simulink model "time_conv_test"  (R2016b)
settings: Solver=VariableStepAuto  StartTime=0.0  StopTime=0  RelTol=1e-3
libraries: GPS_time_lib x1, YMDHMS_2_dec_year x1, time_conversion_lib x1
settings Model: Creator=Taylor  LastModifiedBy=Taylor

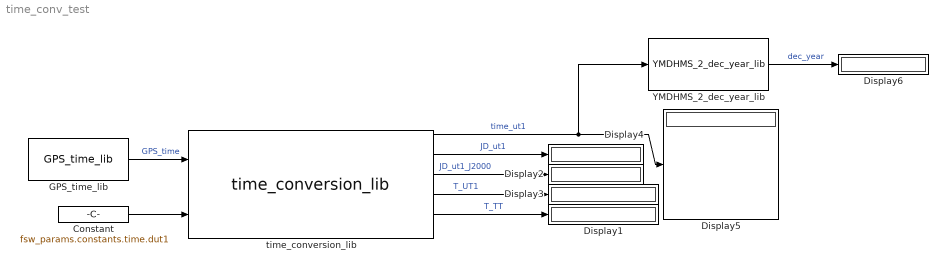
== system time_conv_test ==
  Constant : Constant  Value=fsw_params.constants.time.dut1
  Display{1..6} (6 alike) : Display
  GPS_time_lib : GPS_time_lib/GPS_time_lib
  YMDHMS_2_dec_year_lib : YMDHMS_2_dec_year/YMDHMS_2_dec_year_lib
  time_conversion_lib : time_conversion_lib/time_conversion_lib
  wires:
  GPS_time_lib/1 -> time_conversion_lib/1  "GPS_time"
  time_conversion_lib/3 -> Display2/1  "JD_ut1_J2000"
  time_conversion_lib/4 -> Display3/1  "T_UT1"
  time_conversion_lib/1 -> YMDHMS_2_dec_year_lib/1, Display5/1  "time_ut1"
  YMDHMS_2_dec_year_lib/1 -> Display6/1  "dec_year"
  Constant/1 -> time_conversion_lib/2
  time_conversion_lib/2 -> Display4/1  "JD_ut1"
  time_conversion_lib/5 -> Display1/1  "T_TT"
